simulink model "pi_position_controller"  (R2019a)
settings: Solver=VariableStepAuto  StartTime=0.0  StopTime=inf  RelTol=1e-3
StartFcn:
  | tic;
StopFcn:
  | toc;
undefined symbols (not defined in the file): f, ts
libraries: simulink x1, instrumentlib x1, dspnetwork x1
settings Model: xpc_rtwmakecfg_data=_xpciplib__xpcetherlib__xpcether8255xlib__xpcetherGbElib__xpcnblib_  Creator=Barti  LastModifiedBy=User
settings DataIOCC: ReturnWorkspaceOutputs=off
settings DebuggingCC: ArithmeticOperatorsInVariantConditions=warning
settings SFSimCC: SimUseLocalCustomCode=off
settings RTWCC: RTWUseLocalCustomCode=off
settings CodeAppCC: StateflowObjectComments=on

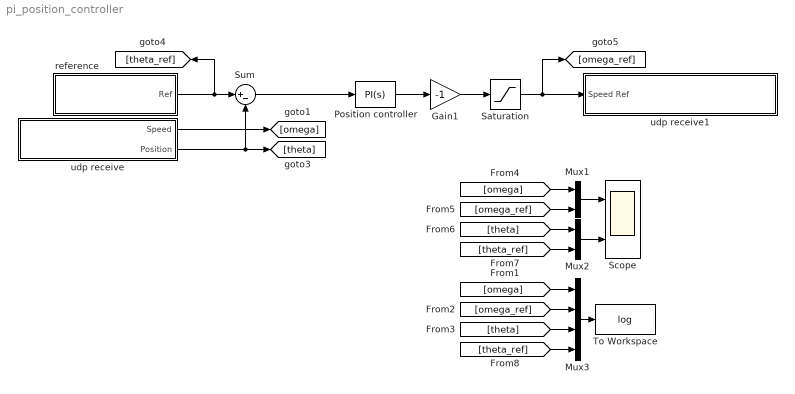
== system pi_position_controller ==
  Gain1 : Gain  Gain=-1
  Mux1 : Mux  Inputs=2
  Mux2 : Mux  Inputs=2
  Mux3 : Mux
  Position controller : simulink/Continuous/PID Controller  Controller=PI  Form=Parallel  TimeDomain=Continuous-time  SampleTime=-1  IntegratorMethod=Forward Euler  FilterMethod=Forward Euler  ControllerParametersSource=internal  P=0.01  I=5  D=0  UseFilter=on  N=100  TunerSelectOption=Transfer Function Based (PID Tuner App)  InitialConditionSource=internal  InitialConditionForIntegrator=0  InitialConditionForFilter=0  DifferentiatorICPrevScaledInput=0  ExternalReset=none  TrackingMode=off  Kt=1  LimitOutput=off  UpperSaturationLimit=inf  LowerSaturationLimit=-inf  LinearizeAsGain=on  AntiWindupMode=none  Kb=1  POutMin=[]  POutMax=[]  IOutMin=[]  IOutMax=[]  DOutMin=[]  DOutMax=[]  NOutMin=[]  NOutMax=[]  SumOutMin=[]  SumOutMax=[]  SaturationOutMin=[]  SaturationOutMax=[]  PParamMin=[]  PParamMax=[]  IParamMin=[]  IParamMax=[]  DParamMin=[]  DParamMax=[]  NParamMin=[]  NParamMax=[]  KbParamMin=[]  KbParamMax=[]  KtParamMin=[]  KtParamMax=[]  KbOutMin=[]  KbOutMax=[]  KtOutMin=[]  KtOutMax=[]  IntegratorOutMin=[]  IntegratorOutMax=[]  FilterOutMin=[]  FilterOutMax=[]  SumI1OutMin=[]  SumI1OutMax=[]  SumI2OutMin=[]  SumI2OutMax=[]  SumI3OutMin=[]  SumI3OutMax=[]  SumI4OutMin=[]  SumI4OutMax=[]  SumDOutMin=[]  SumDOutMax=[]  DifferentiatorOutMin=[]  DifferentiatorOutMax=[]  FilterDiffOutCoefMin=[]  FilterDiffOutCoefMax=[]  ReciprocalOutMin=[]  ReciprocalOutMax=[]  SumDenOutMin=[]  SumDenOutMax=[]  SumNumOutMin=[]  SumNumOutMax=[]  DivideOutMin=[]  DivideOutMax=[]  IntegratorContinuousStateAttributes=''  IntegratorStateMustResolveToSignalObject=off  IntegratorRTWStateStorageClass=Auto  FilterContinuousStateAttributes=''  FilterStateMustResolveToSignalObject=off  FilterRTWStateStorageClass=Auto  ParallelPVariant=InternalParameters  IdealPVariant=Disabled  IVariant=InternalParameters  DVariant=Disabled  IntegratorVariant=Continuous  SatVariant=Disabled  AWVariant=Passthrough  PCopyVariant=Disabled  TRVariant=Disabled  FdbkBlocksVariant=Forward  IdealPFdbkVariant=Disabled  SatFdbkVariant=Disabled  DerivativeFilterVariant=Disabled  NVariant=Disabled  NCopyVariant=Disabled_SignalSpec  FilterICVariant=Disabled  IntegratorICVariant=InternalICs  ExternalResetVariant=Disabled  TRSumVariant=Passthrough  SumFdbkVariant=Disabled  SumVariant=Sum_PI
  Saturation : Saturate  UpperLimit=4500  LowerLimit=-3500
  Scope : Scope  NumInputPorts=2
  Sum : Sum  Inputs=|+-
  To Workspace : ToWorkspace  VariableName=log  SaveFormat=Timeseries  SampleTime=ts
  reference : Subsystem
      mask Display:
      | port_label('output',1,'Ref')
      | fprintf('Random\nsteps')
  udp receive : Subsystem
      mask Display:
      | port_label('output',1,'Speed')
      | port_label('output',2,'Position')
      | fprintf('UDP Receive\n192.168.2.15')
  udp receive1 : Subsystem
      mask Display:
      | port_label('input',1,'Speed Ref')
      | fprintf('UDP Send\n192.168.2.15')
  wires:
  Saturation/1 -> udp receive1/1(Speed Ref), [omega_ref]
  Position controller/1 -> Gain1/1
  Sum/1 -> Position controller/1
  Gain1/1 -> Saturation/1
  reference/1(Ref) -> [theta_ref], Sum/1
  udp receive/2(Position) -> [theta], Sum/2
  udp receive/1(Speed) -> [omega]
  Mux1/1 -> Scope/1
  Mux2/1 -> Scope/2
  [omega] -> Mux1/1
  [omega_ref] -> Mux1/2
  [theta] -> Mux2/1
  [theta_ref] -> Mux2/2
  [theta_ref] -> Mux3/4
  Mux3/1 -> To Workspace/1
  [omega_ref] -> Mux3/2
  [theta] -> Mux3/3
  [omega] -> Mux3/1

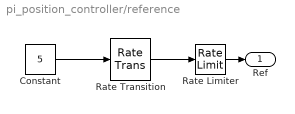
== system pi_position_controller/reference ==
  Constant : Constant  Value=5
  Rate Limiter : RateLimiter  RisingSlewLimit=100  FallingSlewLimit=-100  SampleTimeMode=inherited
  Rate Transition : RateTransition  InitialCondition=-20  OutPortSampleTime=ts
  Ref : Outport
  wires:
  Rate Transition/1 -> Rate Limiter/1
  Constant/1 -> Rate Transition/1
  Rate Limiter/1 -> Ref/1

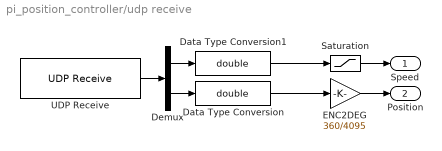
== system pi_position_controller/udp receive ==
  Data Type Conversion : DataTypeConversion  OutDataTypeStr=double
  Data Type Conversion1 : DataTypeConversion  OutDataTypeStr=double
  Demux : Demux  Outputs=2
  ENC2DEG : Gain  Gain=360/4095
  Saturation : Saturate  UpperLimit=4500  LowerLimit=-3500
  UDP Receive : instrumentlib/UDP Receive  Host=192.168.2.15  Port=8889  LocalPort=22000  EnablePortSharing=off  GetLatestData=off  DataSize=2  DataType=int32  ASCIIFormatting=%f,  Terminator=LF  ByteOrder=LittleEndian  EnableBlockingMode=on  Timeout=100  SampleTime=ts  LocalAddress=0.0.0.0
      settings: SourceProductName=Instrument Control Toolbox
  Speed : Outport
  Position : Outport  Port=2
  wires:
  UDP Receive/1 -> Demux/1
  Demux/2 -> Data Type Conversion/1
  Demux/1 -> Data Type Conversion1/1
  ENC2DEG/1 -> Position/1
  Data Type Conversion/1 -> ENC2DEG/1
  Data Type Conversion1/1 -> Saturation/1
  Saturation/1 -> Speed/1

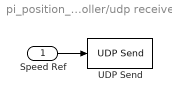
== system pi_position_controller/udp receive1 ==
  Speed Ref : Inport
  UDP Send : dspnetwork/UDP Send  remoteURL='192.168.2.15'  remotePort=8889  localURL='0.0.0.0'  localPortSource=Specify via dialog  localPort=22001  sampletime=-1  blockPlatform=[]  separateLengthPort=0
      settings: SourceProductName=Simulink
  wires:
  Speed Ref/1 -> UDP Send/1
